simulink library "Blocks_Lib"  (R2019b)
settings: Solver=VariableStepAuto  StartTime=0.0  StopTime=10.0  RelTol=1e-3
libraries: simulink x9, $bdroot x9
(part 1 of 2)
settings Model: Creator=aw5670  LastModifiedBy=bhisma
settings DataIOCC: ReturnWorkspaceOutputs=off
settings DebuggingCC: ArithmeticOperatorsInVariantConditions=warning
settings SFSimCC: SimUseLocalCustomCode=off  CustomCodeUndefinedFunction=UseInterfaceOnly
settings RTWCC: RTWUseLocalCustomCode=off
settings CodeAppCC: StateflowObjectComments=on

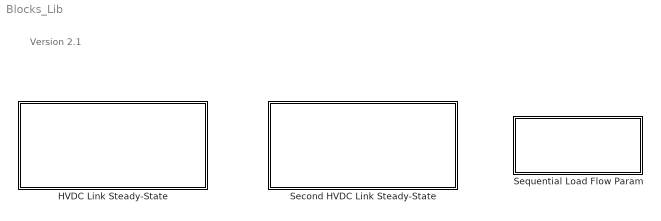
== system Blocks_Lib ==
  note: Version 2.1
  HVDC Link Steady-State : Subsystem  mask(HVDC link steady-state model){NB_R=2, NOT_USED_3=, NOT_USED_4=, Pn_R=600, U1_R=[735, 0.0025, 0.01], U2_R=[200, 0.0025, 0.11], NOT_USED_0=DC current, NOT_USED_1=0, AMODE_ANGLE=5, LOCK_TAP_R=on, TCC_UDI0_MODE_R=off, ANGLE_R=[14.0, 17.0], Udi0_ref_R=280, TSTP_R=0.0125, TAP_R=[0.9375, 1.125], TAP_R_INI=1, Eac_R_INI=735, NB_I=2, NOT_USED_5=, NOT_USED_6=, Pn_I=600, U1_I=[735, 0.0025, 0.01], U2_I=[200, 0.0025, 0.11], C_MODE_I=DC voltage, GAMMA_REF=22, VSCHED=500, GMODE_ANGLE=17, NOT_USED_2=0, LOCK_TAP_I=off, TCC_UDI0_MODE_I=off, ANGLE_I=[20.0, 23.0], Udi0_ref_I=280, TSTP_I=0.0125, TAP_I=[0.9125, 1.0875], TAP_I_INI=1, Eac_I_INI=735, RDC=12.0 + 2*0.3, RCOMP=0.3, MC_MODE=Power, SLACK_ST=Rectifier, SETVAL_MW=1000, SETVAL_kA=2, VCMODE=500*0.94, DELTI=0.2, Tap_pu_R=0.9375, Eac_R=740.8893, Udi0_R=290.4097, Tap_limited_R=0, alpha_R=16.1762, Idc_R=2, Vdc_R=524.6, Pdc_R=1049.2, Pac_R=1054.5333, Qac_R=479.4564, Tap_pu_I=0.975, Eac_I=758.8212, Udi0_I=285.9986, Tap_limited_I=0, alpha_I=144.587, gamma_I=22.8031, Vdc_I=499.4, Pdc_I=-998.8, Pac_I=-993.4667, Qac_I=562.6279, DC_iter=2, Ts=1}
      mask prompts: NB_R "Number of 6 pulse converter units in series"; NOT_USED_3 "AC bus name"; NOT_USED_4 "PQ load name"; Pn_R "Power (MVA)"; U1_R "Primary winding (AC side) parameters [V1 Ph-Ph(kVrms), R1(pu), L1(pu)]"; U2_R "Secondary winding (DC side) parameters [V2 Ph-Ph(kVrms), R2(pu), L2(pu)]"; NOT_USED_0 "Control mode"; NOT_USED_1 "not used"; AMODE_ANGLE "Minimum alpha (deg.)"; LOCK_TAP_R "Lock tap ratio"; TCC_UDI0_MODE_R "Udi0 control mode"; ANGLE_R "Angle range [min, max] (deg.)"; Udi0_ref_R "Udi0 reference (kV)"; TSTP_R "Tap step size (pu)"; TAP_R "Tap range [min, max] (pu)"; TAP_R_INI "Tap ratio (pu)"; Eac_R_INI "Primary AC voltage  (Ph-Ph(kVrms))"; NB_I "Number of 6 pulse converter units in series"; NOT_USED_5 "AC bus name"; NOT_USED_6 "PQ load name"; Pn_I "Power (MVA)"; U1_I "Primary winding (AC side) parameters [V1 Ph-Ph(kVrms), R1(pu), L1(pu)]"; U2_I "Secondary winding (DC side) parameters [V2 Ph-Ph(kVrms), R2(pu), L2(pu)]"; C_MODE_I "Control mode"; GAMMA_REF "Gamma reference (deg.)"; VSCHED "Voltage reference (kV)"; GMODE_ANGLE "Minimum gamma (deg.)"; NOT_USED_2 "Not used"; LOCK_TAP_I "Lock tap ratio"; TCC_UDI0_MODE_I "Udi0 control mode"; ANGLE_I "Angle range  [min, max] (deg.)"; Udi0_ref_I "Udi0 reference (kV)"; TSTP_I "Tap step size (pu)"; TAP_I "Tap range [min, max] (pu)"; TAP_I_INI "Tap ratio (pu)"; Eac_I_INI "Primary AC voltage  (Ph-Ph(kVrms))"; RDC "Total link resistance (ohm)"; RCOMP "Resistance between voltage measurement and converter (ohm)"; MC_MODE "Control mode"; SLACK_ST "Slack station"; SETVAL_MW "Power reference (MW)"; SETVAL_kA "Current reference (kA)"; VCMODE "Inverter DC voltage threshold in power control (kV)"; DELTI "Inverter current margin (kA)"; Tap_pu_R "Tap ratio (pu)"; Eac_R "Eac (kV)"; Udi0_R "Udi0 (kV)"; Tap_limited_R "Tap is limited"; alpha_R "Alpha (deg.)"; Idc_R "Idc (kA)"; Vdc_R "Vdc (kV)"; Pdc_R "Pdc (MW)"; Pac_R "Pac (MW)"; Qac_R "Qac (Mvar)"; Tap_pu_I "Tap ratio (pu)"; Eac_I "Eac (kV)"; Udi0_I "Udi0 (kV)"; Tap_limited_I "Tap is limited"; alpha_I "Alpha (deg.)"; gamma_I "Gamma (deg.)"; Vdc_I "Vdc (kV)"; Pdc_I "Pdc (MW)"; Pac_I "Pac (MW)"; Qac_I "Qac (Mvar)"; DC_iter "Iterations"; Ts "Sample time :"
      mask help: Implements a steady state model of a two terminal HVDC link for the DC load flow solution.
      mask init:
      | % History values 
      | Eac_R     = Eac_R_INI;
      | Eac_I     = Eac_I_INI;
      | TAPINI_R  = TAP_R_INI;
      | TAPINI_I  = TAP_I_INI;
      | 
      | % --- RECTIFIER ---
      | 
      | % Primary
      | V1_R = U1_R(1);
      | R1_R = U1_R(2);
      | L1_R = U1_R(3);
      | 
      | % Secondary
      | V2_R = U2_R(1);
      | R2_R = U2_R(2);
      | L2_R = U2_R(3);
      | 
      | % Nominal turn ratio (Usec/Uprim):
      | TR_R = V2_R/V1_R;
      | 
      | % Transformer reactance seen from secondary, per bridge [XC](ohm):
      | XC_R = (L1_R+L2_R)*V2_R^2/Pn_R;
      | 
      | % Transformer resistance seen from secondary, per bridge [RC](ohm):
      | RC_R = (R1_R+R2_R)* V2_R^2/Pn_R; 
      | 
      | % Tap Changer Control
      | ALFMIN_R=ANGLE_R(1);
      | ALFMAX_R=ANGLE_R(2);
      | 
      | TAPMN_R=TAP_R(1);
      | TAPMX_R=TAP_R(2);
      | 
      | % --- INVERTER ---
      | % Primary
      | V1_I = U1_I(1);
      | R1_I = U1_I(2);
      | L1_I = U1_I(3);
      | 
      | % Secondary
      | V2_I = U2_I(1);
      | R2_I = U2_I(2);
      | L2_I = U2_I(3);
      | 
      | % Nominal turn ratio (Usec/Uprim):
      | TR_I = V2_I/V1_I;
      | 
      | % Transformer reactance seen from secondary, per bridge [XC](ohm):
      | XC_I = (L1_I+L2_I)*V2_I^2/Pn_I;
      | 
      | % Transformer resistance seen from secondary, per bridge [RC](ohm):
      | RC_I = (R1_I+R2_I)* V2_I^2/Pn_I; 
      | 
      | % Pole Control
      | GC = C_MODE_I - 1;  % GC (0/1) is used in the model
      | 
      | % Tap Changer Control
      | GAMMIN_I=ANGLE_I(1);
      | GAMMAX_I=ANGLE_I(2);
      | 
      | TAPMN_I=TAP_I(1);
      | TAPMX_I=TAP_I(2);
      | 
      | DCVMIN_I   = VSCHED * (1 - TSTP_I);     %(kV)
      | DCVMAX_I   = VSCHED * (1 + TSTP_I);
      | 
      | % --- Master Control ---
      | MDC = MC_MODE - 1;     % MDC (0,1, or 2) used in the model 
      | 
      | if (MDC == 1)   
      |     SETVAL = SETVAL_MW;
      | elseif (MDC == 2)
      |     SETVAL = SETVAL_kA;
      | else
      |     SETVAL = 0;
      | end
      mask Help: web('HVDC_Link_SS_help_V2_1.htm');
      mask TypeOptions NOT_USED_0: DC current
      mask Callback LOCK_TAP_R:
      | mode=get_param(gcb,'LOCK_TAP_R');
      | cb = get_param(gcb,'MaskEnables');
      | cb{11}='on'; cb{12}='on';
      | 
      | if strcmp(mode,'on')
      |  cb{11}='off';  % Udi0 control mode
      |  cb{12}='off';  % Angle range
      | end
      | 
      | set_param(gcb,'MaskEnables',cb);
      mask Callback TCC_UDI0_MODE_R:
      | mode=get_param(gcb,'TCC_UDI0_MODE_R');
      | cb = get_param(gcb,'MaskEnables');
      | cb{10}='on'; cb{12}='on'; cb{13}='off';
      | 
      | if strcmp(mode,'on')
      |  cb{12}='off';  % Angle range
      |  cb{10}='off';  % Lock the tap position
      |  cb{13}='on';  % Lock the tap position
      | end
      | 
      | set_param(gcb,'MaskEnables',cb);
      mask TypeOptions C_MODE_I: DC voltage | Gamma angle
      mask Callback C_MODE_I:
      | mode=get_param(gcb,'C_MODE_I');
      | cb = get_param(gcb,'MaskEnables');
      | cb{25}='on'; cb{26}='on'; cb{27}='on'; cb{31}='on';
      | 
      | if strcmp(mode,'Gamma angle')
      |  cb{26}='off';    % Voltage reference
      |  cb{27}='off';    % Minimum gamma
      |  cb{31}='off';    % Angle range (gamma_
      | else
      |  cb{25}='off';    % Gamma reference
      | end
      | 
      | set_param(gcb,'MaskEnables',cb);
      mask Callback LOCK_TAP_I:
      | mode=get_param(gcb,'LOCK_TAP_I');
      | cb = get_param(gcb,'MaskEnables');
      | cb{30}='on'; cb{31}='on';
      | 
      | if strcmp(mode,'on')
      |  cb{30}='off';  % Udi0 control mode
      |  cb{31}='off';  % Angle range
      | end
      | 
      | set_param(gcb,'MaskEnables',cb);
      mask Callback TCC_UDI0_MODE_I:
      | mode=get_param(gcb,'TCC_UDI0_MODE_I');
      | cb = get_param(gcb,'MaskEnables');
      | cb{29}='on'; cb{31}='on';  cb{32}='off';
      | 
      | if strcmp(mode,'on')
      |  cb{29}='off';  % Lock the tap position
      |  cb{31}='off';  % Angle range
      |  cb{32}='on';   % Udi0 reference
      | end
      | 
      | set_param(gcb,'MaskEnables',cb);
      mask TypeOptions MC_MODE: Blocked | Power | Current
      mask Callback MC_MODE:
      | mode=get_param(gcb,'MC_MODE');
      | cb = get_param(gcb,'MaskEnables');
      |  cb{40}='on'; cb{41}='on'; cb{42}='on'; cb{43}='on';
      | 
      | if strcmp(mode,'Current')
      |  cb{40}='off';     % Slack station
      |  cb{41}='off';     % Power reference
      |  cb{43}='off';     % Inverter DC ...
      | end
      | 
      | if strcmp(mode,'Power')
      |  cb{42}='off';     % Current reference
      | end
      | 
      | set_param(gcb,'MaskEnables',cb);
      | clear cb mode;
      mask TypeOptions SLACK_ST: Rectifier | Inverter
      mask DialogControl Container7 Prompt: Rectifier
      mask DialogControl Container10 Prompt: Converter
      mask DialogControl Container14 Prompt: Transformer nominal values per converter unit
      mask DialogControl Container13 Prompt: Control
      mask DialogControl Container16 Prompt: Tap Changer Control
      mask DialogControl Container27 Prompt: Initial values
      mask DialogControl Update_tap_R Prompt: Update
      mask DialogControl Update_tap_R Callback:
      | set_param(gcb,'TAP_R_INI',[num2str(Tap_pu_R(end)), '  %Updated']);
      | 
      | % Reset output values
      | set_param(gcb,'Idc_R',[num2str(0)]);
      | set_param(gcb,'alpha_R',[num2str(0)]);
      | set_param(gcb,'Udi0_R',[num2str(0)]);
      | set_param(gcb,'Vdc_R',[num2str(0)]);
      | set_param(gcb,'Pac_R',[num2str(0)]);
      | set_param(gcb,'Qac_R',[num2str(0)]);
      | set_param(gcb,'Pdc_R',[num2str(0)]);
      mask DialogControl Container12 Prompt: Inverter
      mask DialogControl Container15 Prompt: Converter
      mask DialogControl Container18 Prompt: Transformer nominal values per converter unit
      mask DialogControl Container19 Prompt: Control
      mask DialogControl Container20 Prompt: Tap Changer Control
      mask DialogControl Container28 Prompt: Initial values
      mask DialogControl Update_tap_I Prompt: Update
      mask DialogControl Update_tap_I Callback:
      | set_param(gcb,'TAP_I_INI',[num2str(Tap_pu_I(end)), '  %Updated']);
      | 
      | % Reset output values
      | set_param(gcb,'gamma_I',[num2str(0)]);
      | set_param(gcb,'alpha_I',[num2str(0)]);
      | set_param(gcb,'Udi0_I',[num2str(0)]);
      | set_param(gcb,'Vdc_I',[num2str(0)]);
      | set_param(gcb,'Pdc_I',[num2str(0)]);
      | set_param(gcb,'Pac_I',[num2str(0)]);
      | set_param(gcb,'Qac_I',[num2str(0)]);
      mask DialogControl Container25 Prompt: DC network
      mask DialogControl Container26 Prompt: Master Control
      mask DialogControl Container30 Prompt: Result
      mask DialogControl Container31 Prompt: Rectifier
      mask DialogControl Container33 Prompt: Inverter
      mask DialogControl Control4 Prompt: Compute and Update
      mask DialogControl Control4 Callback:
      | sim(gcs);
      | set_param(gcb,'DC_iter',[num2str(DC_iter(end))]);
      | % Rectifier
      | set_param(gcb,'Eac_R',[num2str(Eac_R(end))]);
      | set_param(gcb,'Tap_pu_R',[num2str(Tap_pu_R(end))]);
      | set_param(gcb,'Tap_limited_R',[num2str(Tap_limited_R(end))]);
      | set_param(gcb,'Idc_R',[num2str(Idc_R(end))]);
      | set_param(gcb,'alpha_R',[num2str(alpha_R(end))]);
      | set_param(gcb,'Udi0_R',[num2str(Udi0_R(end))]);
      | set_param(gcb,'Vdc_R',[num2str(Vdc_R(end))]);
      | set_param(gcb,'Pdc_R',[num2str(Pdc_R(end))]);
      | set_param(gcb,'Pac_R',[num2str(Pac_R(end))]);
      | set_param(gcb,'Qac_R',[num2str(Qac_R(end))]);
      | 
      | % Inverter
      | set_param(gcb,'Eac_I',[num2str(Eac_I(end))]);
      | set_param(gcb,'Tap_pu_I',[num2str(Tap_pu_I(end))]);
      | set_param(gcb,'Tap_limited_I',[num2str(Tap_limited_I(end))]);
      | set_param(gcb,'gamma_I',[num2str(gamma_I(end))]);
      | set_param(gcb,'alpha_I',[num2str(alpha_I(end))]);
      | set_param(gcb,'Udi0_I',[num2str(Udi0_I(end))]);
      | set_param(gcb,'Vdc_I',[num2str(Vdc_I(end))]);
      | set_param(gcb,'Pdc_I',[num2str(Pdc_I(end))]);
      | set_param(gcb,'Pac_I',[num2str(Pac_I(end))]);
      | set_param(gcb,'Qac_I',[num2str(Qac_I(end))]);
      mask Display: disp('Steady-state model\nof HVDC link\n\n(for DC load flow solution)')
  Second HVDC Link Steady-State : Subsystem  mask(HVDC link steady-state model){NB_R=2, NOT_USED_3=, NOT_USED_4=, Pn_R=600, U1_R=[735, 0.0025, 0.01], U2_R=[200, 0.0025, 0.11], NOT_USED_0=DC current, NOT_USED_1=0, AMODE_ANGLE=5, LOCK_TAP_R=off, TCC_UDI0_MODE_R=off, ANGLE_R=[14.0, 17.0], Udi0_ref_R=280, TSTP_R=0.0125, TAP_R=[0.9375, 1.125], TAP_R_INI=1, Eac_R_INI=735, NB_I=2, NOT_USED_5=, NOT_USED_6=, Pn_I=600, U1_I=[735, 0.0025, 0.01], U2_I=[200, 0.0025, 0.11], C_MODE_I=DC voltage, GAMMA_REF=22, VSCHED=500, GMODE_ANGLE=17, NOT_USED_2=0, LOCK_TAP_I=off, TCC_UDI0_MODE_I=off, ANGLE_I=[20.0, 23.0], Udi0_ref_I=280, TSTP_I=0.0125, TAP_I=[0.9125, 1.0875], TAP_I_INI=1, Eac_I_INI=735, RDC=12.0 + 2*0.3, RCOMP=0.3, MC_MODE=Power, SLACK_ST=Rectifier, SETVAL_MW=100, SETVAL_kA=2, VCMODE=500*0.94, DELTI=0.2, Tap_pu_R_B=0.9375, Eac_R_B=740.8893, Udi0_R_B=290.4097, Tap_limited_R_B=0, alpha_R_B=16.1762, Idc_R_B=2, Vdc_R_B=524.6, Pdc_R_B=1049.2, Pac_R_B=1054.5333, Qac_R_B=479.4564, Tap_pu_I_B=0.975, Eac_I_B=758.8212, Udi0_I_B=285.9986, Tap_limited_I_B=0, alpha_I_B=144.587, gamma_I_B=22.8031, Vdc_I_B=499.4, Pdc_I_B=-998.8, Pac_I_B=-993.4667, Qac_I_B=562.6279, DC_iter_B=2, Ts=1}
      mask prompts: NB_R "Number of 6 pulse converter units in series"; NOT_USED_3 "AC bus name"; NOT_USED_4 "PQ load name"; Pn_R "Power (MVA)"; U1_R "Primary winding (AC side) parameters [V1 Ph-Ph(kVrms), R1(pu), L1(pu)]"; U2_R "Secondary winding (DC side) parameters [V2 Ph-Ph(kVrms), R2(pu), L2(pu)]"; NOT_USED_0 "Control mode"; NOT_USED_1 "not used"; AMODE_ANGLE "Minimum alpha (deg.)"; LOCK_TAP_R "Lock tap ratio"; TCC_UDI0_MODE_R "Udi0 control mode"; ANGLE_R "Angle range [min, max] (deg.)"; Udi0_ref_R "Udi0 reference (kV)"; TSTP_R "Tap step size (pu)"; TAP_R "Tap range [min, max] (pu)"; TAP_R_INI "Tap ratio (pu)"; Eac_R_INI "Primary AC voltage  (Ph-Ph(kVrms))"; NB_I "Number of 6 pulse converter units in series"; NOT_USED_5 "AC bus name"; NOT_USED_6 "PQ load name"; Pn_I "Power (MVA)"; U1_I "Primary winding (AC side) parameters [V1 Ph-Ph(kVrms), R1(pu), L1(pu)]"; U2_I "Secondary winding (DC side) parameters [V2 Ph-Ph(kVrms), R2(pu), L2(pu)]"; C_MODE_I "Control mode"; GAMMA_REF "Gamma reference (deg.)"; VSCHED "Voltage reference (kV)"; GMODE_ANGLE "Minimum gamma (deg.)"; NOT_USED_2 "Not used"; LOCK_TAP_I "Lock tap ratio"; TCC_UDI0_MODE_I "Udi0 control mode"; ANGLE_I "Angle range  [min, max] (deg.)"; Udi0_ref_I "Udi0 reference (kV)"; TSTP_I "Tap step size (pu)"; TAP_I "Tap range [min, max] (pu)"; TAP_I_INI "Tap ratio (pu)"; Eac_I_INI "Primary AC voltage  (Ph-Ph(kVrms))"; RDC "Total link resistance (ohm)"; RCOMP "Resistance between voltage measurement and converter (ohm)"; MC_MODE "Control mode"; SLACK_ST "Slack station"; SETVAL_MW "Power reference (MW)"; SETVAL_kA "Current reference (kA)"; VCMODE "Inverter DC voltage threshold in power control (kV)"; DELTI "Inverter current margin (kA)"; Tap_pu_R_B "Tap ratio (pu)"; Eac_R_B "Eac (kV)"; Udi0_R_B "Udi0 (kV)"; Tap_limited_R_B "Tap is limited"; alpha_R_B "Alpha (deg.)"; Idc_R_B "Idc (kA)"; Vdc_R_B "Vdc (kV)"; Pdc_R_B "Pdc (MW)"; Pac_R_B "Pac (MW)"; Qac_R_B "Qac (Mvar)"; Tap_pu_I_B "Tap ratio (pu)"; Eac_I_B "Eac (kV)"; Udi0_I_B "Udi0 (kV)"; Tap_limited_I_B "Tap is limited"; alpha_I_B "Alpha (deg.)"; gamma_I_B "Gamma (deg.)"; Vdc_I_B "Vdc (kV)"; Pdc_I_B "Pdc (MW)"; Pac_I_B "Pac (MW)"; Qac_I_B "Qac (Mvar)"; DC_iter_B "Iterations"; Ts "Sample time :"
      mask help:
      | Implements a steady state model of a two terminal HVDC link  for a DC load flow solution.
      | Note: When using the sequential AC-DC solution methode, the second DC link should be represented by this block.
      mask init:
      | % History values 
      | Eac_R_B     = Eac_R_INI;
      | Eac_I_B     = Eac_I_INI;
      | TAPINI_R_B  = TAP_R_INI;
      | TAPINI_I_B  = TAP_I_INI;
      | 
      | % --- RECTIFIER ---
      | 
      | % Primary
      | V1_R = U1_R(1);
      | R1_R = U1_R(2);
      | L1_R = U1_R(3);
      | 
      | % Secondary
      | V2_R = U2_R(1);
      | R2_R = U2_R(2);
      | L2_R = U2_R(3);
      | 
      | % Nominal turn ratio (Usec/Uprim):
      | TR_R = V2_R/V1_R;
      | 
      | % Transformer reactance seen from secondary, per bridge [XC](ohm):
      | XC_R = (L1_R+L2_R)*V2_R^2/Pn_R;
      | 
      | % Transformer resistance seen from secondary, per bridge [RC](ohm):
      | RC_R = (R1_R+R2_R)* V2_R^2/Pn_R; 
      | 
      | % Tap Changer Control
      | ALFMIN_R=ANGLE_R(1);
      | ALFMAX_R=ANGLE_R(2);
      | 
      | TAPMN_R=TAP_R(1);
      | TAPMX_R=TAP_R(2);
      | 
      | % --- INVERTER ---
      | % Primary
      | V1_I = U1_I(1);
      | R1_I = U1_I(2);
      | L1_I = U1_I(3);
      | 
      | % Secondary
      | V2_I = U2_I(1);
      | R2_I = U2_I(2);
      | L2_I = U2_I(3);
      | 
      | % Nominal turn ratio (Usec/Uprim):
      | TR_I = V2_I/V1_I;
      | 
      | % Transformer reactance seen from secondary, per bridge [XC](ohm):
      | XC_I = (L1_I+L2_I)*V2_I^2/Pn_I;
      | 
      | % Transformer resistance seen from secondary, per bridge [RC](ohm):
      | RC_I = (R1_I+R2_I)* V2_I^2/Pn_I; 
      | 
      | % Pole Control
      | GC = C_MODE_I - 1;  % GC (0/1) is used in the model
      | 
      | % Tap Changer Control
      | GAMMIN_I=ANGLE_I(1);
      | GAMMAX_I=ANGLE_I(2);
      | 
      | TAPMN_I=TAP_I(1);
      | TAPMX_I=TAP_I(2);
      | 
      | DCVMIN_I   = VSCHED * (1 - TSTP_I);     %(kV)
      | DCVMAX_I   = VSCHED * (1 + TSTP_I);
      | 
      | % --- Master Control ---
      | MDC = MC_MODE - 1;     % MDC (0,1, or 2) used in the model 
      | 
      | if (MDC == 1)   
      |     SETVAL = SETVAL_MW;
      | elseif (MDC == 2)
      |     SETVAL = SETVAL_kA;
      | else
      |     SETVAL = 0;
      | end
      mask Help: web('HVDC_Link_SS_help_V2_1.htm');
      mask TypeOptions NOT_USED_0: DC current
      mask Callback LOCK_TAP_R:
      | mode=get_param(gcb,'LOCK_TAP_R');
      | cb = get_param(gcb,'MaskEnables');
      | cb{11}='on'; cb{12}='on';
      | 
      | if strcmp(mode,'on')
      |  cb{11}='off';  % Udi0 control mode
      |  cb{12}='off';  % Angle range
      | end
      | 
      | set_param(gcb,'MaskEnables',cb);
      mask Callback TCC_UDI0_MODE_R:
      | mode=get_param(gcb,'TCC_UDI0_MODE_R');
      | cb = get_param(gcb,'MaskEnables');
      | cb{10}='on'; cb{12}='on'; cb{13}='off';
      | 
      | if strcmp(mode,'on')
      |  cb{12}='off';  % Angle range
      |  cb{10}='off';  % Lock the tap position
      |  cb{13}='on';  % Lock the tap position
      | end
      | 
      | set_param(gcb,'MaskEnables',cb);
      mask TypeOptions C_MODE_I: DC voltage | Gamma angle
      mask Callback C_MODE_I:
      | mode=get_param(gcb,'C_MODE_I');
      | cb = get_param(gcb,'MaskEnables');
      | cb{25}='on'; cb{26}='on'; cb{27}='on'; cb{31}='on';
      | 
      | if strcmp(mode,'Gamma angle')
      |  cb{26}='off';    % Voltage reference
      |  cb{27}='off';    % Minimum gamma
      |  cb{31}='off';    % Angle range (gamma_
      | else
      |  cb{25}='off';    % Gamma reference
      | end
      | 
      | set_param(gcb,'MaskEnables',cb);
      mask Callback LOCK_TAP_I:
      | mode=get_param(gcb,'LOCK_TAP_I');
      | cb = get_param(gcb,'MaskEnables');
      | cb{30}='on'; cb{31}='on';
      | 
      | if strcmp(mode,'on')
      |  cb{30}='off';  % Udi0 control mode
      |  cb{31}='off';  % Angle range
      | end
      | 
      | set_param(gcb,'MaskEnables',cb);
      mask Callback TCC_UDI0_MODE_I:
      | mode=get_param(gcb,'TCC_UDI0_MODE_I');
      | cb = get_param(gcb,'MaskEnables');
      | cb{29}='on'; cb{31}='on';  cb{32}='off';
      | 
      | if strcmp(mode,'on')
      |  cb{29}='off';  % Lock the tap position
      |  cb{31}='off';  % Angle range
      |  cb{32}='on';   % Udi0 reference
      | end
      | 
      | set_param(gcb,'MaskEnables',cb);
      mask TypeOptions MC_MODE: Blocked | Power | Current
      mask Callback MC_MODE:
      | mode=get_param(gcb,'MC_MODE');
      | cb = get_param(gcb,'MaskEnables');
      |  cb{40}='on'; cb{41}='on'; cb{42}='on'; cb{43}='on';
      | 
      | if strcmp(mode,'Current')
      |  cb{40}='off';     % Slack station
      |  cb{41}='off';     % Power reference
      |  cb{43}='off';     % Inverter DC ...
      | end
      | 
      | if strcmp(mode,'Power')
      |  cb{42}='off';     % Current reference
      | end
      | 
      | set_param(gcb,'MaskEnables',cb);
      | clear cb mode;
      mask TypeOptions SLACK_ST: Rectifier | Inverter
      mask DialogControl Container7 Prompt: Rectifier
      mask DialogControl Container10 Prompt: Converter
      mask DialogControl Container14 Prompt: Transformer nominal values per converter unit
      mask DialogControl Container13 Prompt: Control
      mask DialogControl Container16 Prompt: Tap Changer Control
      mask DialogControl Container27 Prompt: Initial values
      mask DialogControl Update_tap_R Prompt: Update
      mask DialogControl Update_tap_R Callback:
      | set_param(gcb,'TAP_R_INI',[num2str(Tap_pu_R(end)), '  %Updated']);
      | 
      | % Reset output values
      | set_param(gcb,'Idc_R',[num2str(0)]);
      | set_param(gcb,'alpha_R',[num2str(0)]);
      | set_param(gcb,'Udi0_R',[num2str(0)]);
      | set_param(gcb,'Vdc_R',[num2str(0)]);
      | set_param(gcb,'Pac_R',[num2str(0)]);
      | set_param(gcb,'Qac_R',[num2str(0)]);
      | set_param(gcb,'Pdc_R',[num2str(0)]);
      mask DialogControl Container12 Prompt: Inverter
      mask DialogControl Container15 Prompt: Converter
      mask DialogControl Container18 Prompt: Transformer nominal values per converter unit
      mask DialogControl Container19 Prompt: Control
      mask DialogControl Container20 Prompt: Tap Changer Control
      mask DialogControl Container28 Prompt: Initial values
      mask DialogControl Update_tap_I Prompt: Update
      mask DialogControl Update_tap_I Callback:
      | set_param(gcb,'TAP_I_INI',[num2str(Tap_pu_I(end)), '  %Updated']);
      | 
      | % Reset output values
      | set_param(gcb,'gamma_I',[num2str(0)]);
      | set_param(gcb,'alpha_I',[num2str(0)]);
      | set_param(gcb,'Udi0_I',[num2str(0)]);
      | set_param(gcb,'Vdc_I',[num2str(0)]);
      | set_param(gcb,'Pdc_I',[num2str(0)]);
      | set_param(gcb,'Pac_I',[num2str(0)]);
      | set_param(gcb,'Qac_I',[num2str(0)]);
      mask DialogControl Container25 Prompt: DC network
      mask DialogControl Container26 Prompt: Master Control
      mask DialogControl Container30 Prompt: Result
      mask DialogControl Container31 Prompt: Rectifier
      mask DialogControl Container33 Prompt: Inverter
      mask DialogControl Control4 Prompt: Compute and Update
      mask DialogControl Control4 Callback:
      | sim(gcs);
      | set_param(gcb,'DC_iter_B',[num2str(DC_iter_B(end))]);
      | % Rectifier
      | set_param(gcb,'Eac_R_B',[num2str(Eac_R_B(end))]);
      | set_param(gcb,'Tap_pu_R_B',[num2str(Tap_pu_R_B(end))]);
      | set_param(gcb,'Tap_limited_R_B',[num2str(Tap_limited_R_B(end))]);
      | set_param(gcb,'Idc_R_B',[num2str(Idc_R_B(end))]);
      | set_param(gcb,'alpha_R_B',[num2str(alpha_R_B(end))]);
      | set_param(gcb,'Udi0_R_B',[num2str(Udi0_R_B(end))]);
      | set_param(gcb,'Vdc_R_B',[num2str(Vdc_R_B(end))]);
      | set_param(gcb,'Pdc_R_B',[num2str(Pdc_R_B(end))]);
      | set_param(gcb,'Pac_R_B',[num2str(Pac_R_B(end))]);
      | set_param(gcb,'Qac_R_B',[num2str(Qac_R_B(end))]);
      | 
      | % Inverter
      | set_param(gcb,'Eac_I_B',[num2str(Eac_I_B(end))]);
      | set_param(gcb,'Tap_pu_I_B',[num2str(Tap_pu_I_B(end))]);
      | set_param(gcb,'Tap_limited_I_B',[num2str(Tap_limited_I_B(end))]);
      | set_param(gcb,'gamma_I_B',[num2str(gamma_I_B(end))]);
      | set_param(gcb,'alpha_I_B',[num2str(alpha_I_B(end))]);
      | set_param(gcb,'Udi0_I_B',[num2str(Udi0_I_B(end))]);
      | set_param(gcb,'Vdc_I_B',[num2str(Vdc_I_B(end))]);
      | set_param(gcb,'Pdc_I_B',[num2str(Pdc_I_B(end))]);
      | set_param(gcb,'Pac_I_B',[num2str(Pac_I_B(end))]);
      | set_param(gcb,'Qac_I_B',[num2str(Qac_I_B(end))]);
      mask Display: disp('Steady-state model\nof HVDC link\n\n(for DC load flow solution)')
  Sequential Load Flow Param : Subsystem  mask(Parameters for the sequential AC-DC load flow algorithm){Set_original=on, Model_network=LF_AC29bus_HVDCdemo_V2_1, DC_max_iter=10, DC_AC_max=10, LFDClink=Link_A, Report=ACDC_report_A.txt, bus_rec=LG27, Load_rec=LG27_DC, bus_inv=MTL7, Load_inv=MTL7_DC, second_link=off, LFDClink_B=Link_B, Report_B=ACDC_report_B.txt, bus_rec_B=LG27, Load_rec_B=North-West Network/LG27_DC_B, bus_inv_B=MTL7, load_inv_B=MTL7_DC_B, Start_LF=off}
      mask prompts: Set_original "Reset original work space"; Model_network "AC-DC network model name"; DC_max_iter "Maximum iterations for DC load flow solution"; DC_AC_max "Maximum sequential AC-DC load flows"; LFDClink "DC link steady-state model name"; Report "DC link load flow report name"; bus_rec "Rectifier AC bus name"; Load_rec "PQ load name (Rectifier)"; bus_inv "Inverter AC bus name"; Load_inv "PQ load name (Inverter)"; second_link "Second DC link present"; LFDClink_B "Second DC link steady-state model name"; Report_B "Second DC link load flow report name"; bus_rec_B "Second rectifier AC bus name"; Load_rec_B "PQ load name (Second rectifier)"; bus_inv_B "Second inverter AC bus name"; load_inv_B "PQ load name (Second inverter)"; Start_LF "Start"
      mask help:
      | The block specifies the parameters used by the script  LF_ACDC_solve_V2_1
      | solving by the sequential algorithm the load flow of an AC network that
      | includes one or two HVDC links.  The script is called by the 'Compute' button.
      mask Help: web('Sequential_LF_param_help.htm');
      mask Callback second_link:
      | mode=get_param(gcb,'second_link');
      | cb = get_param(gcb,'MaskEnables');
      | cb{12}='off';cb{13}='off';cb{14}='off';
      | cb{15}='off';cb{16}='off';cb{17}='off';
      | 
      | if strcmp(mode,'on')
      |  cb{12}='on';     % Second DC link model name
      |  cb{13}='on';     % Second DC link report name
      |  cb{14}='on';     % Second rectifier AC bus ...
      |  cb{15}='on';     % PQ load name (second rectifier)
      |  cb{16}='on';     % Second rectifier AC bus ...
      |  cb{17}='on';     % PQ load name (second inverter)
      | end
      | 
      | set_param(gcb,'MaskEnables',cb);
      mask Callback Start_LF:
      | mode=get_param(gcb,'Start_LF');
      | cb = get_param(gcb,'MaskEnables');
      | cb{17}='on';
      | 
      | if strcmp(mode,'on')
      | 
      |  %LF_ACDC_solve_V2b
      |  10
      | end
      | 
      | set_param(gcb,'start_LF','off');
      mask DialogControl Container8 Prompt: Sequential Load flow
      mask DialogControl Execute_LF Prompt: Compute
      mask DialogControl Execute_LF Callback:
      | clear cb mode;
      | eval('LF_ACDC_solve_V2_1');
      mask DialogControl Container6 Prompt: DC link
      mask DialogControl Container29 Prompt: Second DC link
      mask Display: disp('Sequential AC-DC\nload flow\nparameters')

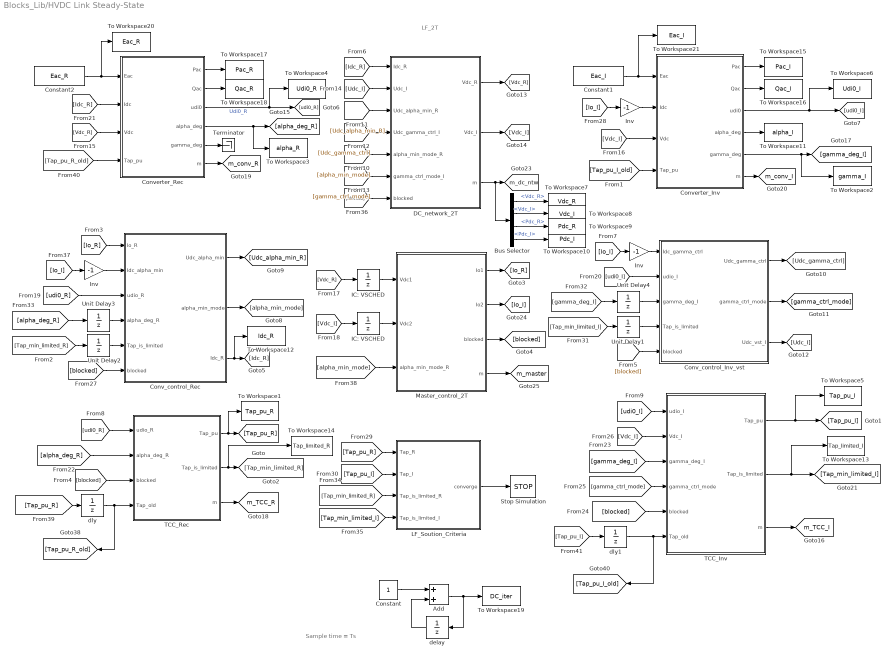
== system Blocks_Lib/HVDC Link Steady-State ==
  note: LF_2T
  note: Sample time = Ts
  " Inv " : Gain  Gain=-1
  Add : Sum
  Bus Selector : BusSelector  OutputSignals=Vdc_R,Vdc_I,Pdc_R,Pdc_I
  Constant : Constant
  Constant1 : Constant  Value=Eac_I
  Constant2 : Constant  Value=Eac_R
  Conv_control_Inv_vst : Subsystem  mask(Converter controls - voltage setting inverter){GC=GC, VSCHED=VSCHED, GMODE_ANGLE=GMODE_ANGLE, GAMMA_REF=GAMMA_REF, NB=NB_I, RC=RC_I, XC=XC_I}
      mask prompts: GC "Gamma control mode [GC] (1/0):"; VSCHED "Scheduled dc voltage [VSCHED] (kV):"; GMODE_ANGLE "Gamma minimum mode angle [GMODE_ANGLE] (deg):"; GAMMA_REF "Gamma reference angle [GAMMA_REF] (deg):"; NB "Number of 6 pulse bridges in series [NB]:"; RC "Resistance seen from secondary, per bridge [RC] (ohm):"; XC "Reactance seen from secondary, per bridge [XC] (ohm):"
  Conv_control_Rec : Subsystem  mask(Converter controls - Rectifier){AMODE_ANGLE=AMODE_ANGLE, NB=NB_R, RC=RC_R, XC=XC_R}
      mask prompts: AMODE_ANGLE "Alpha minimum mode angle   [AMODE_ANGLE] (deg):"; NB "Number of 6 pulse bridges in series [NB]:"; RC "Resistance seen from secondary, per bridge [RC] (ohm):"; XC "Reactance seen from secondary, per bridge [XC] (ohm):"
      settings: MinAlgLoopOccurrences=on
  Converter_Inv : Subsystem  mask(Converter unit data - Inverter){Pn=Pn_I, W1=[V1_I,  R1_I,  L1_I], W2=[V2_I, R2_I, L2_I], TR=V2_I/V1_I, RC=(R1_I+R2_I)* V2_I^2/Pn_I;, XC=(L1_I+L2_I)*V2_I^2/Pn_I;, NB=NB_I}
      mask prompts: Pn "One bridge, Transformer Nominal power [Pn(MVA)]:"; W1 "Primary winding (AC side) [V1 Ph-Ph(kVrms), R1(pu), L1(pu)]:"; W2 "Secondary winding (DC side) [V2 Ph-Ph(kVrms), R2 (pu), L2(pu)]:"; TR "Nominal turn ratio (Usec/Uprim) [TR] (pu):"; RC "Resistance seen from secondary, per bridge [RC] (ohm):"; XC "Reactance seen from secondary, per bridge [XC] (ohm):"; NB "Number of 6p bridges in series [NB]:"
  Converter_Rec : Subsystem  mask(Converter unit data - Rectifier){Pn=Pn_R, W1=[V1_R,  R1_R,  L1_R], W2=[V2_R,  R2_R,  L2_R], TR=V2_R/V1_R, RC=(R1_R+R2_R)* V2_R^2/Pn_R;, XC=(L1_R+L2_R)*V2_R^2/Pn_R;, NB=NB_R}
      mask prompts: Pn "One bridge, Transformer Nominal power [Pn(MVA)]:"; W1 "Primary winding (AC side) [V1 Ph-Ph(kVrms), R1(pu), L1(pu)]:"; W2 "Secondary winding (DC side) [V2 Ph-Ph(kVrms), R2 (pu), L2(pu)]:"; TR "Nominal turn ratio (Usec/Uprim) [TR] (pu):"; RC "Resistance seen from secondary, per bridge [RC] (ohm):"; XC "Reactance seen from secondary, per bridge [XC] (ohm):"; NB "Number of 6p bridges in series [NB]:"
  DC_network_2T : Subsystem  mask(DC network - 2 terminals){RDC=RDC, RCOMP=RCOMP}
      mask prompts: RDC "DC network resistance [RDC] (ohm):"; RCOMP "Compensating resistance for voltage control [RCOMP] (ohm):"
  IC: VSCHED : UnitDelay  InitialCondition=VSCHED  SampleTime=-1  HasFrameUpgradeWarning=on
  "IC: VSCHED " : UnitDelay  InitialCondition=VSCHED  SampleTime=-1  HasFrameUpgradeWarning=on
  "Inv " : Gain  Gain=-1
  "Inv  " : Gain  Gain=-1
  LF_Soution_Criteria : Subsystem
  Master_control_2T : Subsystem  mask(Master control for 3 terminals (RMCC)){MDC=MDC, SLACK_ST=SLACK_ST, SETVAL=SETVAL, VCMODE=VCMODE}
      mask prompts: MDC "Control mode [MDC] (0,1,2):"; SLACK_ST "Slack station [SLACK_ST] (1,2):"; SETVAL "Desired power or current [SETVAL] (MW or kA):"; VCMODE "Minimum DC voltage for power control [VCMODE] (kV):"
      mask help:
      | - The slack station (1, 2 or 3) will compensate for the DC network losses.
      | - Desired power or current: negative at inverter; positive at rectifier (sum shoud be zero).
  Stop Simulation : Stop
  TCC_Inv : Subsystem  mask(Tap Change Control (TCC) at the inverter){LOCK_TAP=LOCK_TAP_I, TCC_UDI0_MODE=TCC_UDI0_MODE_I, Udi0_ref=Udi0_ref_I, TAPINI=TAPINI_I, TAPMN=TAPMN_I, TAPMX=TAPMX_I, TSTP=TSTP_I, GAMMIN=GAMMIN_I, GAMMAX=GAMMAX_I, DCVMIN=DCVMIN_I, DCVMAX=DCVMAX_I}
      mask prompts: LOCK_TAP "Lock tap position at initial value [LOCK_TAP] (1/0):"; TCC_UDI0_MODE "TC in UDI0 control mode (around Udi0_ref) [TCC_UDI0_MODE] (1/0):"; Udi0_ref "Reference Udi0 voltage [Udi0_ref] (KV):"; TAPINI "Initial Tap ratio  [TAPINI] (pu):"; TAPMN "Minimum tap ratio [TAPMN] (pu):"; TAPMX "Maximum tap ratio [TAPMX] (pu):"; TSTP "Transformer tap-step [TSTP] (pu):"; GAMMIN "Minimum margin  (gamma) angle [GAMMIN] (deg):"; GAMMAX "Maximum margin  (gamma) angle [GAMMAX] (deg):"; DCVMIN "Minimum DC voltage [DCVMIN] (kV):"; DCVMAX "Maximum DC voltage [DCVMAX] (kV):"
      mask init:
      | Udi0_min = (1-TSTP*0.75)* Udi0_ref;  % kV
      | Udi0_max = (1+TSTP*0.75)* Udi0_ref;
      settings: AttributesFormatString=|
      | Udi0_min = (1-TSTP*0.75)* Udi0_ref
      | Udi0_max = (1+TSTP*0.75)* Udi0_ref
  TCC_Rec : Subsystem  mask(Tap Change Control (TCC) at the rectifier){LOCK_TAP=LOCK_TAP_R, TCC_UDI0_MODE=TCC_UDI0_MODE_R, Udi0_ref=Udi0_ref_R, TAPINI=TAPINI_R, TAPMN=TAPMN_R, TAPMX=TAPMX_R, TSTP=TSTP_R, ALFMIN=ALFMIN_R, ALFMAX=ALFMAX_R}
      mask prompts: LOCK_TAP "Lock tap position at initial value [LOCK_TAP] (1/0):"; TCC_UDI0_MODE "TC in UDI0 control mode (around Udi0_ref) [TCC_UDI0_MODE] (1/0):"; Udi0_ref "Reference Udi0 voltage [Udi0_ref] (KV):"; TAPINI "Initial Tap ratio  [TAPINI] (pu):"; TAPMN "Minimum tap ratio [TAPMN] (pu):"; TAPMX "Maximum tap ratio [TAPMX] (pu):"; TSTP "Transformer tap-step [TSTP] (pu):"; ALFMIN "Minimum firing (alpha) angle [ALFMIN] (deg):"; ALFMAX "Maximum firing (alpha) angle [ALFMAX] (deg):"
      mask init:
      | Udi0_min = (1-TSTP*0.75)* Udi0_ref;  % kV
      | Udi0_max = (1+TSTP*0.75)* Udi0_ref;
      settings: AttributesFormatString=|
      | Udi0_min = (1-TSTP*0.75)* Udi0_ref
      | Udi0_max = (1+TSTP*0.75)* Udi0_ref
  Terminator : Terminator
  To Workspace1 : ToWorkspace  VariableName=Tap_pu_R  SampleTime=-1
  To Workspace10 : ToWorkspace  VariableName=Pdc_I  SampleTime=-1
  To Workspace11 : ToWorkspace  VariableName=alpha_I  SampleTime=-1
  To Workspace12 : ToWorkspace  VariableName=Idc_R  SampleTime=-1
  To Workspace13 : ToWorkspace  VariableName=Tap_limited_I  SampleTime=-1
  To Workspace14 : ToWorkspace  VariableName=Tap_limited_R  SampleTime=-1
  To Workspace15 : ToWorkspace  VariableName=Pac_I  SampleTime=-1
  To Workspace16 : ToWorkspace  VariableName=Qac_I  SampleTime=-1
  To Workspace17 : ToWorkspace  VariableName=Pac_R  SampleTime=-1
  To Workspace18 : ToWorkspace  VariableName=Qac_R  SampleTime=-1
  To Workspace19 : ToWorkspace  VariableName=DC_iter  SampleTime=-1
  To Workspace2 : ToWorkspace  VariableName=gamma_I  SampleTime=-1
  To Workspace20 : ToWorkspace  VariableName=Eac_R  SampleTime=-1
  To Workspace21 : ToWorkspace  VariableName=Eac_I  SampleTime=-1
  To Workspace3 : ToWorkspace  VariableName=alpha_R  SampleTime=-1
  To Workspace4 : ToWorkspace  VariableName=Udi0_R  SampleTime=-1
  To Workspace5 : ToWorkspace  VariableName=Tap_pu_I  SampleTime=-1
  To Workspace6 : ToWorkspace  VariableName=Udi0_I  SampleTime=-1
  To Workspace7 : ToWorkspace  VariableName=Vdc_R  SampleTime=-1
  To Workspace8 : ToWorkspace  VariableName=Vdc_I  SampleTime=-1
  To Workspace9 : ToWorkspace  VariableName=Pdc_R  SampleTime=-1
  Unit Delay{1..4} (4 alike) : UnitDelay  SampleTime=-1  HasFrameUpgradeWarning=on
  delay : UnitDelay  SampleTime=Ts  HasFrameUpgradeWarning=on
      settings: AttributesFormatString=IC=%<InitialCondition>
  dly : UnitDelay  InitialCondition=TAPINI_R  SampleTime=-1  HasFrameUpgradeWarning=on
      settings: AttributesFormatString=IC=%<InitialCondition>
  dly1 : UnitDelay  InitialCondition=TAPINI_I  SampleTime=-1  HasFrameUpgradeWarning=on
      settings: AttributesFormatString=IC=%<InitialCondition>
  tag scope: m_TCC_I=global, m_TCC_R=global, m_conv_I=global, m_conv_R=global, m_dc_ntw=global, m_master=global
  wires:
  Constant1/1 -> Converter_Inv/1(Eac), To Workspace21/1
  Constant2/1 -> Converter_Rec/1(Eac), To Workspace20/1
  delay/1 -> Add/2
  Constant/1 -> Add/1
  Add/1 -> delay/1, To Workspace19/1
  [alpha_deg_R] -> TCC_Rec/2(alpha_deg_R)
  [Tap_pu_I] -> dly1/1
  dly1/1 -> TCC_Inv/6(Tap_old), [Tap_pu_I_old]
  [Tap_pu_R] -> dly/1
  dly/1 -> TCC_Rec/4(Tap_old), [Tap_pu_R_old]
  [gamma_deg_I] -> Unit Delay4/1
  Unit Delay4/1 -> Conv_control_Inv_vst/3(gamma_deg_I)
  Unit Delay3/1 -> Conv_control_Rec/4(alpha_deg_R)
  [alpha_deg_R] -> Unit Delay3/1
  Unit Delay2/1 -> Conv_control_Rec/5(Tap_is_limited)
  [Tap_min_limited_R] -> Unit Delay2/1
  Bus Selector/2 -> To Workspace8/1  "<Vdc_I>"
  Bus Selector/3 -> To Workspace9/1  "<Pdc_R>"
  Bus Selector/4 -> To Workspace10/1  "<Pdc_I>"
  Bus Selector/1 -> To Workspace7/1  "<Vdc_R>"
  [Tap_pu_I_old] -> Converter_Inv/4(Tap_pu)
  [Io_I] -> " Inv "/1
  [udi0_R] -> Conv_control_Rec/3(udio_R)
  [blocked] -> Conv_control_Rec/6(blocked)
  [blocked] -> DC_network_2T/7(blocked)
  [Tap_min_limited_I] -> LF_Soution_Criteria/4(Tap_is_limited_I)
  [Tap_min_limited_R] -> LF_Soution_Criteria/3(Tap_is_limited_R)
  [Tap_pu_I] -> LF_Soution_Criteria/2(Tap_I)
  TCC_Rec/3(m) -> [m_TCC_R]
  TCC_Rec/1(Tap_pu) -> [Tap_pu_R], To Workspace1/1
  TCC_Inv/3(m) -> [m_TCC_I]
  Unit Delay1/1 -> Conv_control_Inv_vst/4(Tap_is_limited)
  [blocked] -> Conv_control_Inv_vst/5(blocked)
  [Tap_min_limited_I] -> Unit Delay1/1
  Converter_Inv/2(Qac) -> To Workspace16/1
  Converter_Inv/1(Pac) -> To Workspace15/1
  Converter_Rec/2(Qac) -> To Workspace18/1
  Converter_Rec/1(Pac) -> To Workspace17/1
  [Tap_pu_R] -> LF_Soution_Criteria/1(Tap_R)
  Converter_Inv/6(m) -> [m_conv_I]
  Converter_Rec/6(m) -> [m_conv_R]
  [Vdc_I] -> Converter_Inv/3(Vdc)
  Converter_Rec/5(gamma_deg) -> Terminator/1
  [Vdc_I] -> TCC_Inv/2(Vdc_I)
  [gamma_ctrl_mode] -> TCC_Inv/4(gamma_ctrl_mode)
  [blocked] -> TCC_Inv/5(blocked)
  [gamma_deg_I] -> TCC_Inv/3(gamma_deg_I)
  Converter_Inv/5(gamma_deg) -> To Workspace2/1, [gamma_deg_I]
  Converter_Inv/4(alpha_deg) -> To Workspace11/1
  Converter_Rec/4(alpha_deg) -> [alpha_deg_R], To Workspace3/1
  [Idc_R] -> Converter_Rec/2(Idc)
  [udi0_I] -> Conv_control_Inv_vst/2(udio_I)
  [Vdc_I] -> "IC: VSCHED "/1
  [Vdc_R] -> IC: VSCHED/1
  [Vdc_R] -> Converter_Rec/3(Vdc)
  DC_network_2T/2(Vdc_I) -> [Vdc_I]
  DC_network_2T/1(Vdc_R) -> [Vdc_R]
  [Udc_I] -> DC_network_2T/2(Udc_I)
  Conv_control_Inv_vst/3(Udc_vst_I) -> [Udc_I]
  [gamma_ctrl_mode] -> DC_network_2T/6(gamma_ctrl_mode_I)
  Conv_control_Inv_vst/2(gamma_ctrl_mode) -> [gamma_ctrl_mode]
  [Udc_gamma_ctrl] -> DC_network_2T/4(Udc_gamma_ctrl_I)
  Conv_control_Inv_vst/1(Udc_gamma_ctrl) -> [Udc_gamma_ctrl]
  [Udc_alpha_min_R] -> DC_network_2T/3(Udc_alpha_min_R)
  Conv_control_Rec/1(Udc_alpha_min) -> [Udc_alpha_min_R]
  [alpha_min_mode] -> DC_network_2T/5(alpha_min_mode_R)
  Conv_control_Rec/2(alpha_min_mode) -> [alpha_min_mode]
  [Tap_pu_R_old] -> Converter_Rec/4(Tap_pu)
  [udi0_I] -> TCC_Inv/1(udio_I)
  [udi0_R] -> TCC_Rec/1(udio_R)
  Converter_Inv/3(udi0) -> [udi0_I], To Workspace6/1
  Converter_Rec/3(udi0) -> [udi0_R], To Workspace4/1  "Udi0_R"
  [Idc_R] -> DC_network_2T/1(Idc_R)
  [blocked] -> TCC_Rec/3(blocked)
  [Io_R] -> Conv_control_Rec/1(Io_R)
  TCC_Rec/2(Tap_is_limited) -> [Tap_min_limited_R], To Workspace14/1
  TCC_Inv/2(Tap_is_limited) -> [Tap_min_limited_I], To Workspace13/1
  TCC_Inv/1(Tap_pu) -> [Tap_pu_I], To Workspace5/1
  "IC: VSCHED "/1 -> Master_control_2T/2(Vdc2)
  IC: VSCHED/1 -> Master_control_2T/1(Vdc1)
  [alpha_min_mode] -> Master_control_2T/3(alpha_min_mode_R)
  Master_control_2T/1(Io1) -> [Io_R]
  Master_control_2T/2(Io2) -> [Io_I]
  Master_control_2T/3(blocked) -> [blocked]
  Master_control_2T/4(m) -> [m_master]
  "Inv "/1 -> Conv_control_Inv_vst/1(Idc_gamma_ctrl)
  [Io_I] -> "Inv "/1
  "Inv  "/1 -> Converter_Inv/2(Idc)
  [Io_I] -> "Inv  "/1
  DC_network_2T/3(m) -> [m_dc_ntw], Bus Selector/1
  " Inv "/1 -> Conv_control_Rec/2(Idc_alpha_min)
  Conv_control_Rec/3(Idc_R) -> [Idc_R], To Workspace12/1
  LF_Soution_Criteria/1(converge) -> Stop Simulation/1

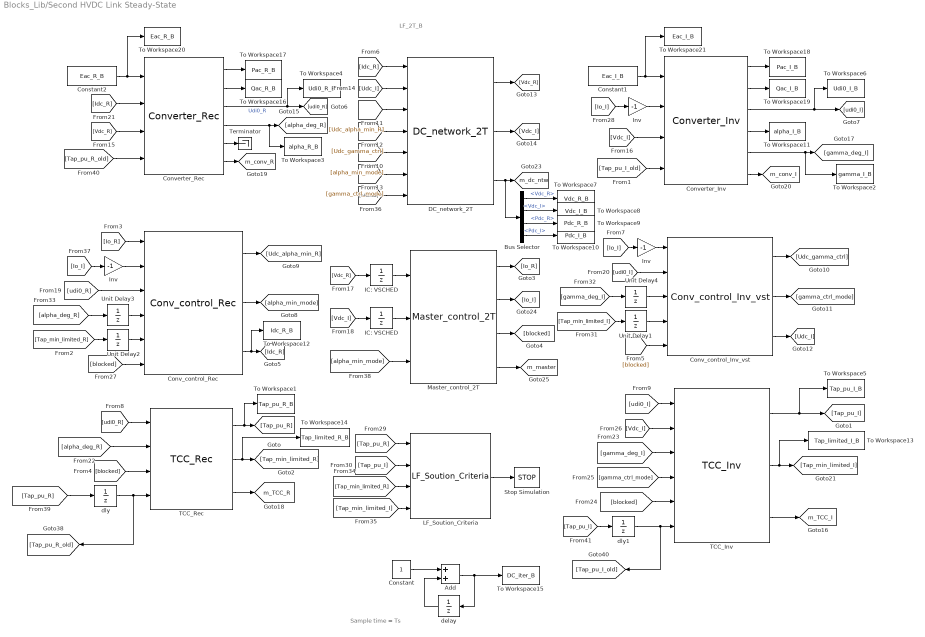
== system Blocks_Lib/Second HVDC Link Steady-State ==
  note: Sample time = Ts
  note: LF_2T_B
  " Inv " : Gain  Gain=-1
  Add : Sum
  Bus Selector : BusSelector  OutputSignals=Vdc_R,Vdc_I,Pdc_R,Pdc_I
  Constant : Constant
  Constant1 : Constant  Value=Eac_I_B
  Constant2 : Constant  Value=Eac_R_B
  Conv_control_Inv_vst : $bdroot/Second HVDC Link Steady-State/Conv_control_Inv_vst  GC=GC  VSCHED=VSCHED  GMODE_ANGLE=GMODE_ANGLE  GAMMA_REF=GAMMA_REF  NB=NB_I  RC=RC_I  XC=XC_I
  Conv_control_Rec : $bdroot/Second HVDC Link Steady-State/Conv_control_Rec  AMODE_ANGLE=AMODE_ANGLE  NB=NB_R  RC=RC_R  XC=XC_R
  Converter_Inv : $bdroot/Second HVDC Link Steady-State/Converter_Inv  Pn=Pn_I  W1="[V1_I,  R1_I,  L1_I]"  W2=[V2_I, R2_I, L2_I]  TR=V2_I/V1_I  RC=(R1_I+R2_I)* V2_I^2/Pn_I;  XC=(L1_I+L2_I)*V2_I^2/Pn_I;  NB=NB_I
  Converter_Rec : $bdroot/Second HVDC Link Steady-State/Converter_Rec  Pn=Pn_R  W1="[V1_R,  R1_R,  L1_R]"  W2="[V2_R,  R2_R,  L2_R]"  TR=V2_R/V1_R  RC=(R1_R+R2_R)* V2_R^2/Pn_R;  XC=(L1_R+L2_R)*V2_R^2/Pn_R;  NB=NB_R
  DC_network_2T : $bdroot/Second HVDC Link Steady-State/DC_network_2T  RDC=RDC  RCOMP=RCOMP
  IC: VSCHED : UnitDelay  InitialCondition=VSCHED  SampleTime=-1  HasFrameUpgradeWarning=on
  "IC: VSCHED " : UnitDelay  InitialCondition=VSCHED  SampleTime=-1  HasFrameUpgradeWarning=on
  "Inv " : Gain  Gain=-1
  "Inv  " : Gain  Gain=-1
  LF_Soution_Criteria : $bdroot/Second HVDC Link Steady-State/LF_Soution_Criteria
  Master_control_2T : $bdroot/Second HVDC Link Steady-State/Master_control_2T  MDC=MDC  SLACK_ST=SLACK_ST  SETVAL=SETVAL  VCMODE=VCMODE
  Stop Simulation : Stop
  TCC_Inv : $bdroot/Second HVDC Link Steady-State/TCC_Inv  LOCK_TAP=LOCK_TAP_I  TCC_UDI0_MODE=TCC_UDI0_MODE_I  Udi0_ref=Udi0_ref_I  TAPINI=TAPINI_I_B  TAPMN=TAPMN_I  TAPMX=TAPMX_I  TSTP=TSTP_I  GAMMIN=GAMMIN_I  GAMMAX=GAMMAX_I  DCVMIN=DCVMIN_I  DCVMAX=DCVMAX_I
      settings: AttributesFormatString=|
      | Udi0_min = (1-TSTP*0.75)* Udi0_ref
      | Udi0_max = (1+TSTP*0.75)* Udi0_ref
  TCC_Rec : $bdroot/Second HVDC Link Steady-State/TCC_Rec  LOCK_TAP=LOCK_TAP_R  TCC_UDI0_MODE=TCC_UDI0_MODE_R  Udi0_ref=Udi0_ref_R  TAPINI=TAPINI_R_B  TAPMN=TAPMN_R  TAPMX=TAPMX_R  TSTP=TSTP_R  ALFMIN=ALFMIN_R  ALFMAX=ALFMAX_R
      settings: AttributesFormatString=|
      | Udi0_min = (1-TSTP*0.75)* Udi0_ref
      | Udi0_max = (1+TSTP*0.75)* Udi0_ref
  Terminator : Terminator
  To Workspace1 : ToWorkspace  VariableName=Tap_pu_R_B  SampleTime=-1
  To Workspace10 : ToWorkspace  VariableName=Pdc_I_B  SampleTime=-1
  To Workspace11 : ToWorkspace  VariableName=alpha_I_B  SampleTime=-1
  To Workspace12 : ToWorkspace  VariableName=Idc_R_B  SampleTime=-1
  To Workspace13 : ToWorkspace  VariableName=Tap_limited_I_B  SampleTime=-1
  To Workspace14 : ToWorkspace  VariableName=Tap_limited_R_B  SampleTime=-1
  To Workspace15 : ToWorkspace  VariableName=DC_iter_B  SampleTime=-1
  To Workspace16 : ToWorkspace  VariableName=Qac_R_B  SampleTime=-1
  To Workspace17 : ToWorkspace  VariableName=Pac_R_B  SampleTime=-1
  To Workspace18 : ToWorkspace  VariableName=Pac_I_B  SampleTime=-1
  To Workspace19 : ToWorkspace  VariableName=Qac_I_B  SampleTime=-1
  To Workspace2 : ToWorkspace  VariableName=gamma_I_B  SampleTime=-1
  To Workspace20 : ToWorkspace  VariableName=Eac_R_B  SampleTime=-1
  To Workspace21 : ToWorkspace  VariableName=Eac_I_B  SampleTime=-1
  To Workspace3 : ToWorkspace  VariableName=alpha_R_B  SampleTime=-1
  To Workspace4 : ToWorkspace  VariableName=Udi0_R_B  SampleTime=-1
  To Workspace5 : ToWorkspace  VariableName=Tap_pu_I_B  SampleTime=-1
  To Workspace6 : ToWorkspace  VariableName=Udi0_I_B  SampleTime=-1
  To Workspace7 : ToWorkspace  VariableName=Vdc_R_B  SampleTime=-1
  To Workspace8 : ToWorkspace  VariableName=Vdc_I_B  SampleTime=-1
  To Workspace9 : ToWorkspace  VariableName=Pdc_R_B  SampleTime=-1
  Unit Delay{1..4} (4 alike) : UnitDelay  SampleTime=-1  HasFrameUpgradeWarning=on
  delay : UnitDelay  SampleTime=Ts  HasFrameUpgradeWarning=on
      settings: AttributesFormatString=IC=%<InitialCondition>
  dly : UnitDelay  InitialCondition=TAPINI_R_B  SampleTime=-1  HasFrameUpgradeWarning=on
      settings: AttributesFormatString=IC=%<InitialCondition>
  dly1 : UnitDelay  InitialCondition=TAPINI_I_B  SampleTime=-1  HasFrameUpgradeWarning=on
      settings: AttributesFormatString=IC=%<InitialCondition>
  tag scope: m_TCC_I=global, m_TCC_R=global, m_conv_I=global, m_conv_R=global, m_dc_ntw=global, m_master=global
  wires:
  delay/1 -> Add/2
  Constant/1 -> Add/1
  Add/1 -> delay/1, To Workspace15/1
  Constant1/1 -> Converter_Inv/1, To Workspace21/1
  Constant2/1 -> Converter_Rec/1, To Workspace20/1
  [alpha_deg_R] -> TCC_Rec/2
  [Tap_pu_I] -> dly1/1
  dly1/1 -> TCC_Inv/6, [Tap_pu_I_old]
  [Tap_pu_R] -> dly/1
  dly/1 -> TCC_Rec/4, [Tap_pu_R_old]
  [gamma_deg_I] -> Unit Delay4/1
  Unit Delay4/1 -> Conv_control_Inv_vst/3
  Unit Delay3/1 -> Conv_control_Rec/4
  [alpha_deg_R] -> Unit Delay3/1
  Unit Delay2/1 -> Conv_control_Rec/5
  [Tap_min_limited_R] -> Unit Delay2/1
  Bus Selector/2 -> To Workspace8/1  "<Vdc_I>"
  Bus Selector/3 -> To Workspace9/1  "<Pdc_R>"
  Bus Selector/4 -> To Workspace10/1  "<Pdc_I>"
  Bus Selector/1 -> To Workspace7/1  "<Vdc_R>"
  [Tap_pu_I_old] -> Converter_Inv/4
  [Io_I] -> " Inv "/1
  [udi0_R] -> Conv_control_Rec/3
  [blocked] -> Conv_control_Rec/6
  [blocked] -> DC_network_2T/7
  LF_Soution_Criteria/1 -> Stop Simulation/1
  [Tap_min_limited_I] -> LF_Soution_Criteria/4
  [Tap_min_limited_R] -> LF_Soution_Criteria/3
  [Tap_pu_I] -> LF_Soution_Criteria/2
  TCC_Rec/3 -> [m_TCC_R]
  TCC_Rec/1 -> [Tap_pu_R], To Workspace1/1
  TCC_Inv/3 -> [m_TCC_I]
  Unit Delay1/1 -> Conv_control_Inv_vst/4
  [blocked] -> Conv_control_Inv_vst/5
  [Tap_min_limited_I] -> Unit Delay1/1
  Converter_Inv/2 -> To Workspace19/1
  Converter_Inv/1 -> To Workspace18/1
  Converter_Rec/2 -> To Workspace16/1
  Converter_Rec/1 -> To Workspace17/1
  [Tap_pu_R] -> LF_Soution_Criteria/1
  Converter_Inv/6 -> [m_conv_I]
  Converter_Rec/6 -> [m_conv_R]
  [Vdc_I] -> Converter_Inv/3
  Converter_Rec/5 -> Terminator/1
  [Vdc_I] -> TCC_Inv/2
  [gamma_ctrl_mode] -> TCC_Inv/4
  [blocked] -> TCC_Inv/5
  [gamma_deg_I] -> TCC_Inv/3
  Converter_Inv/5 -> To Workspace2/1, [gamma_deg_I]
  Converter_Inv/4 -> To Workspace11/1
  Converter_Rec/4 -> [alpha_deg_R], To Workspace3/1
  [Idc_R] -> Converter_Rec/2
  [udi0_I] -> Conv_control_Inv_vst/2
  [Vdc_I] -> "IC: VSCHED "/1
  [Vdc_R] -> IC: VSCHED/1
  [Vdc_R] -> Converter_Rec/3
  DC_network_2T/2 -> [Vdc_I]
  DC_network_2T/1 -> [Vdc_R]
  [Udc_I] -> DC_network_2T/2
  Conv_control_Inv_vst/3 -> [Udc_I]
  [gamma_ctrl_mode] -> DC_network_2T/6
  Conv_control_Inv_vst/2 -> [gamma_ctrl_mode]
  [Udc_gamma_ctrl] -> DC_network_2T/4
  Conv_control_Inv_vst/1 -> [Udc_gamma_ctrl]
  [Udc_alpha_min_R] -> DC_network_2T/3
  Conv_control_Rec/1 -> [Udc_alpha_min_R]
  [alpha_min_mode] -> DC_network_2T/5
  Conv_control_Rec/2 -> [alpha_min_mode]
  [Tap_pu_R_old] -> Converter_Rec/4
  [udi0_I] -> TCC_Inv/1
  [udi0_R] -> TCC_Rec/1
  Converter_Inv/3 -> [udi0_I], To Workspace6/1
  Converter_Rec/3 -> [udi0_R], To Workspace4/1  "Udi0_R"
  [Idc_R] -> DC_network_2T/1
  [blocked] -> TCC_Rec/3
  [Io_R] -> Conv_control_Rec/1
  TCC_Rec/2 -> To Workspace14/1, [Tap_min_limited_R]
  TCC_Inv/2 -> To Workspace13/1, [Tap_min_limited_I]
  TCC_Inv/1 -> [Tap_pu_I], To Workspace5/1
  "IC: VSCHED "/1 -> Master_control_2T/2
  IC: VSCHED/1 -> Master_control_2T/1
  [alpha_min_mode] -> Master_control_2T/3
  Master_control_2T/1 -> [Io_R]
  Master_control_2T/2 -> [Io_I]
  Master_control_2T/3 -> [blocked]
  Master_control_2T/4 -> [m_master]
  "Inv "/1 -> Conv_control_Inv_vst/1
  [Io_I] -> "Inv "/1
  "Inv  "/1 -> Converter_Inv/2
  [Io_I] -> "Inv  "/1
  DC_network_2T/3 -> [m_dc_ntw], Bus Selector/1
  " Inv "/1 -> Conv_control_Rec/2
  Conv_control_Rec/3 -> [Idc_R], To Workspace12/1

== system Blocks_Lib/Sequential Load Flow Param ==

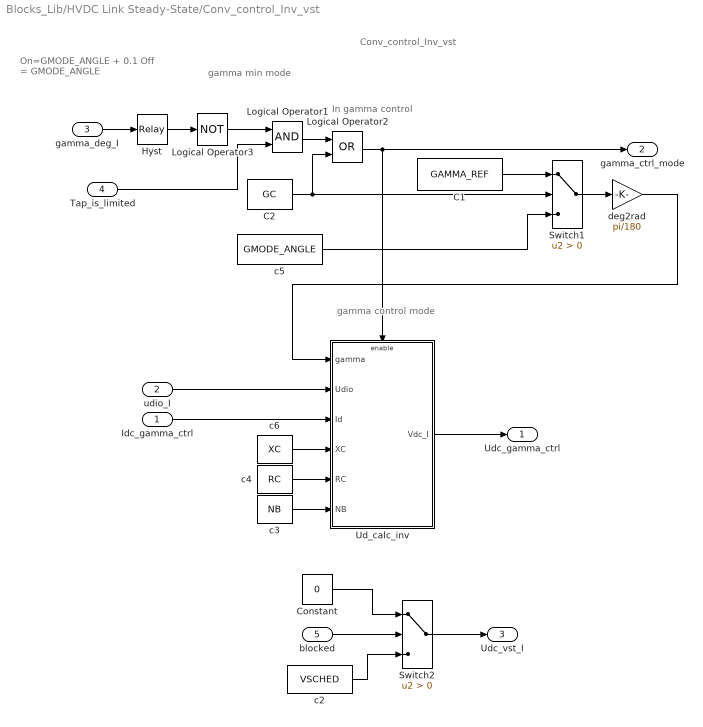
== system Blocks_Lib/HVDC Link Steady-State/Conv_control_Inv_vst ==
  note: gamma min mode
  note: On=GMODE_ANGLE + 0.1
      | Off = GMODE_ANGLE
  note: In gamma control
  note: gamma control mode
  note: Conv_control_Inv_vst
  Idc_gamma_ctrl : Inport
  udio_I : Inport  Port=2
  gamma_deg_I : Inport  Port=3
  Tap_is_limited : Inport  Port=4
  blocked : Inport  Port=5
  C1 : Constant  Value=GAMMA_REF
  C2 : Constant  Value=GC
  Constant : Constant  Value=0
  Hyst : Relay  OnSwitchValue=GMODE_ANGLE + 0.1  OffSwitchValue=GMODE_ANGLE
  Logical Operator1 : Logic  AllPortsSameDT=off  OutDataTypeStr=boolean
  Logical Operator2 : Logic  Operator=OR  AllPortsSameDT=off  OutDataTypeStr=boolean
  Logical Operator3 : Logic  Operator=NOT  AllPortsSameDT=off  OutDataTypeStr=boolean
  Switch1 : Switch  Criteria=u2 > Threshold
  Switch2 : Switch  Criteria=u2 > Threshold
  Ud_calc_inv : Subsystem
  c2 : Constant  Value=VSCHED
  c3 : Constant  Value=NB
  c4 : Constant  Value=RC
  c5 : Constant  Value=GMODE_ANGLE
  c6 : Constant  Value=XC
  deg2rad : Gain  Gain=pi/180
  Udc_gamma_ctrl : Outport
  gamma_ctrl_mode : Outport  Port=2
  Udc_vst_I : Outport  Port=3
  wires:
  Logical Operator3/1 -> Logical Operator1/1
  Hyst/1 -> Logical Operator3/1
  gamma_deg_I/1 -> Hyst/1
  Logical Operator2/1 -> gamma_ctrl_mode/1, Ud_calc_inv/Enable
  deg2rad/1 -> Ud_calc_inv/1(gamma)
  c5/1 -> Switch1/3
  C2/1 -> Logical Operator2/2, Switch1/2
  Logical Operator1/1 -> Logical Operator2/1
  c2/1 -> Switch2/3
  blocked/1 -> Switch2/2
  Constant/1 -> Switch2/1
  Switch2/1 -> Udc_vst_I/1
  Ud_calc_inv/1(Vdc_I) -> Udc_gamma_ctrl/1
  Idc_gamma_ctrl/1 -> Ud_calc_inv/3(Id)
  udio_I/1 -> Ud_calc_inv/2(Udio)
  c6/1 -> Ud_calc_inv/4(XC)
  c4/1 -> Ud_calc_inv/5(RC)
  c3/1 -> Ud_calc_inv/6(NB)
  C1/1 -> Switch1/1
  Switch1/1 -> deg2rad/1
  Tap_is_limited/1 -> Logical Operator1/2
